simulink model "PTHS"  (R2020a)
settings: Solver=FixedStepAuto  StartTime=0.0  StopTime=10.0  FixedStep=1e-3  RelTol=1e-3  EnableMultiTasking=on
undefined symbols (not defined in the file): D0, D1, D10, D11, D12, D13, D2, D3, D4, D5, D6, D7, D8, D9, PTA0, PTA1, PTA2, PTB23, PTB9, PTC16, PTC17, PTC2, PTC3, PTC4, PTD0, PTD1, PTD2, PTD3
libraries: frdmk64flib x14
settings Model: ExtModeTrigDuration=5  Creator=iceca  LastModifiedBy=iceca
settings OptimizationCC: EnhancedBackFolding=on  PassReuseOutputArgsAs=Individual arguments  ZeroExternalMemoryAtStartup=off  ZeroInternalMemoryAtStartup=off  MaxStackSize=64  OptimizeBlockOrder=speed  DifferentSizesBufferReuse=on  OptimizationCustomize=off  EfficientTunableParamExpr=on
settings DebuggingCC: ParameterTunabilityLossMsg=error
settings HardwareCC: ProdBitPerPointer=32  ProdBitPerSizeT=32  ProdBitPerPtrDiffT=32  ProdLargestAtomicInteger=Long  ProdLargestAtomicFloat=Double  ProdWordSize=32  ProdHWDeviceType=ARM Compatible->ARM Cortex
settings SFSimCC: MATLABDynamicMemAlloc=off
settings RTWCC: SystemTargetFile=ert.tlc  HardwareBoard=NXP FRDM-K64F  TemplateMakefile=ert_default_tmf  Toolchain=GNU Tools for ARM Embedded Processors
settings CodeAppCC: ForceParamTrailComments=on  IgnoreCustomStorageClasses=off  OperatorAnnotations=on  SimulinkDataObjDesc=on  SFDataObjDesc=on  InsertBlockDesc=on

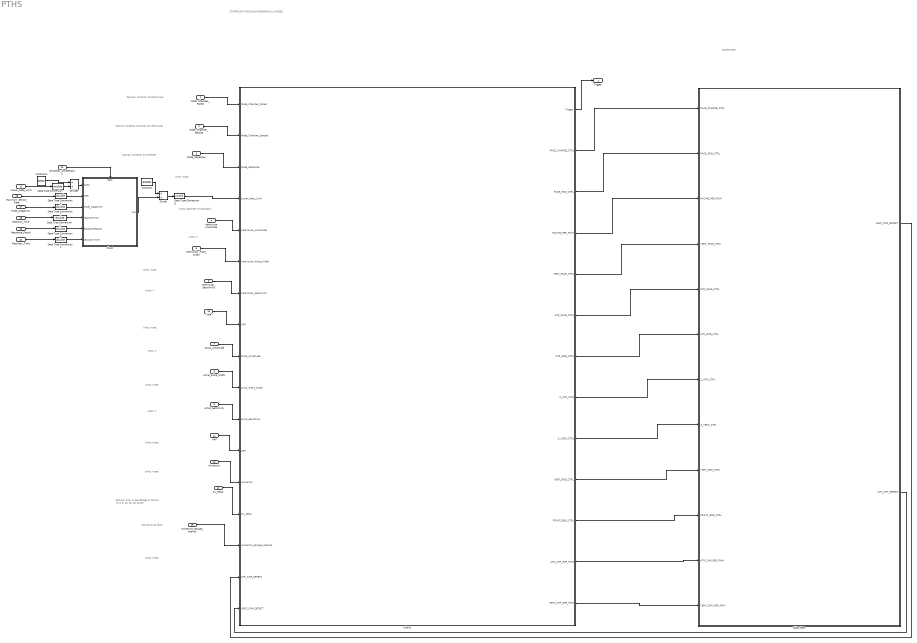
== system PTHS ==
  note: STATEFLOW: PACING and SENSING ALL MODES
  note: Units: msec
  note: Domain:true, false
  note: Domain: 0=None, 1=Atrial, 2=Ventricular
  note: Units: msec
  note: Units: V
  note: Units: V
  note: Units: msec
  note: Domain: OFF, or percentage
      | in the set (3, 6, 9, 12, 15, 18, 21,25)
  note: Units: msec
  note: Units: pace per minute(ppm)
  note: Units: msec
  note: Units: msec
  note: Domain: 1=Atrial, 2=Ventricular
  note: Units: V
  note: Units: msec
  note: Units: V
  note: HARDWARE
  note: Domain: 0=None, 2=Inhibited
  Mode_Chamber_Paced : Inport  OutDataTypeStr=uint8
  Mode_Chamber_Sensed : Inport  Port=2  OutDataTypeStr=uint8
  Mode_Response : Inport  Port=3  OutDataTypeStr=uint8
  Ventricular Amplitude : Inport  Port=4  OutDataTypeStr=uint8
  Ventricular_Pulse_Width : Inport  Port=5  OutDataTypeStr=uint16
  Ventricular_Sensiitivity : Inport  Port=6  OutDataTypeStr=uint8
  Atrial_Amplitude : Inport  Port=7  OutDataTypeStr=uint8
  Atrial_Pulse_Width : Inport  Port=8  OutDataTypeStr=uint16
  Atrial_Sensitivity : Inport  Port=9  OutDataTypeStr=uint8
  Hysterisis : Inport  Port=10  OutDataTypeStr=uint8
  Lower_Rate_Limit : Inport  Port=11  OutDataTypeStr=uint16
  AV_Delay : Inport  Port=12  OutDataTypeStr=uint16
  VRP : Inport  Port=13  OutDataTypeStr=uint16
  ARP : Inport  Port=14  OutDataTypeStr=uint16
  Hysterisis_Escape_Interval : Inport  Port=15  OutDataTypeStr=uint16
  Maximum_Sensor_Rate : Inport  Port=16  OutDataTypeStr=uint8
  Mode_Adaptivity : Inport  Port=17  OutDataTypeStr=uint8
  Reaction_Time : Inport  Port=18  OutDataTypeStr=uint8
  Response_Factor : Inport  Port=19  OutDataTypeStr=uint8
  Recovery_Time : Inport  Port=20  OutDataTypeStr=uint8
  Smoother_Acceleration : Inport  Port=21
  Chart : Stateflow chart  TreatAsAtomicUnit=on
      settings: PortSchema="{\"entries\":[{\"content\":{\"sides\":[{\"content\":{\"connectorIds\":[\"In6\"]},\"type\":\"ConnectorPlacement.EquallySpacedRectSide\",\"uuid\":\"5e590210-4b26-43ca-b410-899265592776\"},{\"content\":{\"connectorIds\":[],\"side\":\"RIGHT\"},\"type\":\"ConnectorPlacement.EquallySpacedRectSide\",\"uuid\":\"99d9f5d1-b5a6-4f8b-b4f2-efe260ebc8c4\"},{\"content\":{\"connectorIds\":[\"Out1\"],\"side\":\"TOP\"},\"type\":\"ConnectorPlacement.EquallySpacedRectSide\",\"uuid\":\"3c56162d-1f91-43ab-bf8d-9a1cf5be554c\"},{\"content\":{\"connectorIds\":[\"In1\",\"In2\",\"In7\",\"In4\",\"In3\",\"In5\"],\"side\":\"BOTTOM\"},\"type\":\"ConnectorPlacement.EquallySpacedRectSide\",\"uuid\":\"2e827a33-e1bf-40db-bbb6-314ece1f4eba\"}]},\"type\":\"ConnectorPlacement.EquallySpacedConnector\",\"uuid\":\"7a7dbe64-1607-48a8-bc2e-dcaf5b987588\"}],\"packageUris\":[\"http://schema.mathworks.com/mf0/Connector/19700101\"],\"version\":\"1.0\"}"
  Chart1 : Stateflow chart  TreatAsAtomicUnit=on
      settings: PortSchema="{\"entries\":[{\"content\":{\"sides\":[{\"content\":{\"connectorIds\":[\"In1\",\"In2\",\"In3\",\"In4\",\"In5\",\"In6\",\"In7\",\"In8\",\"In9\",\"In10\",\"In11\",\"In12\",\"In13\",\"In17\",\"In14\",\"In15\",\"In16\"]},\"type\":\"ConnectorPlacement.EquallySpacedRectSide\",\"uuid\":\"ef801456-a3d3-4c00-800f-18f55ff1f97a\"},{\"content\":{\"connectorIds\":[\"Out1\",\"Out2\",\"Out3\",\"Out4\",\"Out5\",\"Out6\",\"Out7\",\"Out8\",\"Out9\",\"Out10\",\"Out11\",\"Out12\",\"Out13\"],\"side\":\"RIGHT\"},\"type\":\"ConnectorPlacement.EquallySpacedRectSide\",\"uuid\":\"5ac52b61-bf48-4a4b-86f3-012ecfccb962\"},{\"content\":{\"connectorIds\":[],\"side\":\"TOP\"},\"type\":\"ConnectorPlacement.EquallySpacedRectSide\",\"uuid\":\"b91e78a1-d42c-4358-92cf-ad767f596c0a\"}]},\"type\":\"ConnectorPlacement.EquallySpacedConnector\",\"uuid\":\"810cd47a-6ba0-4b6e-85f5-59d182ca7955\"}],\"packageUris\":[\"http://schema.mathworks.com/mf0/Connector/19700101\"],\"version\":\"1.0\"}"
  Constant : Constant  Value=60000  SampleTime=-1
  Constant1 : Constant  Value=60000  SampleTime=-1
  Data Type Conversion{1..5,7} (6 alike) : DataTypeConversion  OutDataTypeStr=double
  Data Type Conversion8 : DataTypeConversion  OutDataTypeStr=uint16
  Divide : Product  Inputs=*/
  Divide1 : Product  Inputs=*/
  Subsystem : Subsystem
  Trigger : Outport
  wires:
  Chart1/1(Trigger) -> Trigger/1
  AV_Delay/1 -> Chart1/17(AV_Delay)
  Chart1/10(VENT_GND_CTRL) -> Subsystem/9(VENT_GND_CTRL)
  Chart1/12(ATR_CMP_REF_PWM) -> Subsystem/11(ATR_CMP_REF_PWM)
  Ventricular_Sensiitivity/1 -> Chart1/7(Ventricular_Sensitivity)
  Hysterisis_Escape_Interval/1 -> Chart1/14(Hysterisis_Escape_Interval)
  Chart1/5(VENT_PACE_CTRL) -> Subsystem/4(VENT_PACE_CTRL)
  Ventricular Amplitude/1 -> Chart1/5(Ventricular_Amplitude)
  VRP/1 -> Chart1/8(VRP)
  Chart1/13(VENT_CMP_REF_PWM) -> Subsystem/12(VENT_CMP_REF_PWM)
  Atrial_Amplitude/1 -> Chart1/9(Atrial_Amplitude)
  Chart1/6(ATR_PACE_CTRL) -> Subsystem/5(ATR_PACE_CTRL)
  Chart1/2(PACE_CHARGE_CTRL) -> Subsystem/1(PACE_CHARGE_CTRL)
  Atrial_Sensitivity/1 -> Chart1/11(Atrial_Sensitivity)
  Atrial_Pulse_Width/1 -> Chart1/10(Atrial_Pulse_Width)
  Mode_Response/1 -> Chart1/3(Mode_Response)
  Chart1/7(ATR_GND_CTRL) -> Subsystem/6(ATR_GND_CTRL)
  Mode_Chamber_Paced/1 -> Chart1/1(Mode_Chamber_Paced)
  Subsystem/1(VENT_CMP_DETECT) -> Chart1/15(ATR_CMP_DETECT)
  Chart1/11(FRONT_END_CTRL) -> Subsystem/10(FRONT_END_CTRL)
  Chart1/8(Z_ATR_CTRL) -> Subsystem/7(Z_ATR_CTRL)
  Chart1/3(PACE_GND_CTRL) -> Subsystem/2(PACE_GND_CTRL)
  Subsystem/2(ATR_CMP_DETECT) -> Chart1/16(VENT_CMP_DETECT)
  ARP/1 -> Chart1/12(ARP)
  Ventricular_Pulse_Width/1 -> Chart1/6(Ventricular_Pulse_Width)
  Mode_Chamber_Sensed/1 -> Chart1/2(Mode_Chamber_Sensed)
  Chart1/9(Z_VENT_CTRL) -> Subsystem/8(Z_VENT_CTRL)
  Chart1/4(PACING_REF_PWM) -> Subsystem/3(PACING_REF_PWM)
  Hysterisis/1 -> Chart1/13(Hysterisis)
  Chart/1(LRL) -> Divide/2
  Lower_Rate_Limit/1 -> Data Type Conversion5/1
  Reaction_Time/1 -> Data Type Conversion2/1
  Data Type Conversion1/1 -> Chart/5(recoveryTime)
  Data Type Conversion7/1 -> Chart/7(Mode_Adaptivity)
  Data Type Conversion2/1 -> Chart/4(reactionTime)
  Constant/1 -> Divide/1
  Data Type Conversion5/1 -> Divide1/2
  Data Type Conversion8/1 -> Chart1/4(Lower_Rate_Limit)
  Mode_Adaptivity/1 -> Data Type Conversion7/1
  Data Type Conversion3/1 -> Chart/3(ResponseFactor)
  Divide/1 -> Data Type Conversion8/1
  Constant1/1 -> Divide1/1
  Divide1/1 -> Chart/1(OLRL)
  Data Type Conversion4/1 -> Chart/2(MSR)
  Response_Factor/1 -> Data Type Conversion3/1
  Recovery_Time/1 -> Data Type Conversion1/1
  Maximum_Sensor_Rate/1 -> Data Type Conversion4/1
  Smoother_Acceleration/1 -> Chart/6(data)

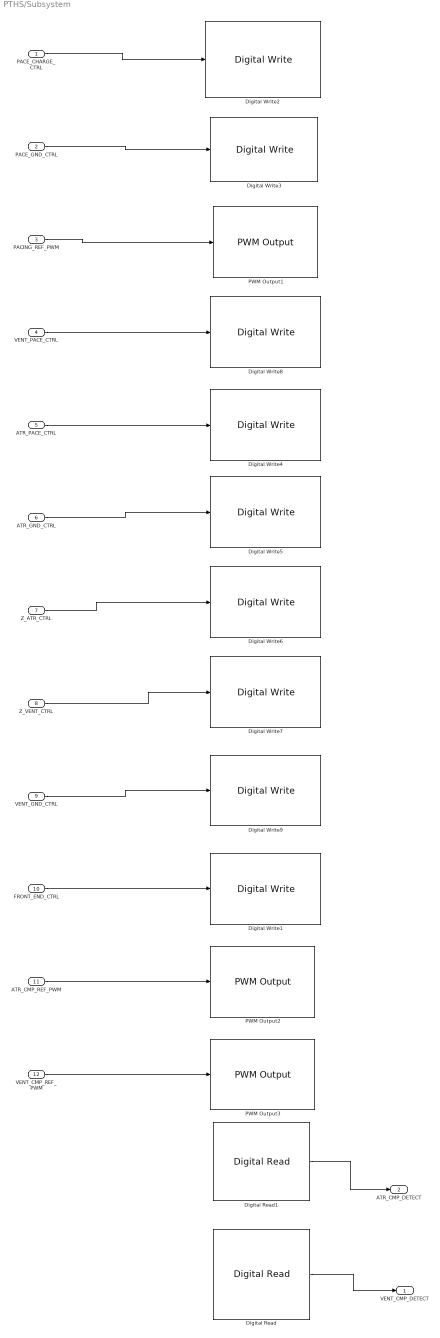
== system PTHS/Subsystem ==
  PACE_CHARGE_CTRL : Inport
  PACE_GND_CTRL : Inport  Port=2
  PACING_REF_PWM : Inport  Port=3
  VENT_PACE_CTRL : Inport  Port=4
  ATR_PACE_CTRL : Inport  Port=5
  ATR_GND_CTRL : Inport  Port=6
  Z_ATR_CTRL : Inport  Port=7
  Z_VENT_CTRL : Inport  Port=8
  VENT_GND_CTRL : Inport  Port=9
  FRONT_END_CTRL : Inport  Port=10
  ATR_CMP_REF_PWM : Inport  Port=11
  VENT_CMP_REF_PWM : Inport  Port=12
  Digital Read : frdmk64flib/Digital Read  Whichpin=PTC16 (D0)  SampleTime=-1
  Digital Read1 : frdmk64flib/Digital Read  Whichpin=PTC17 (D1)  SampleTime=-1
  Digital Write1 : frdmk64flib/Digital Write  Whichpin=PTD1 (D13)
  Digital Write2 : frdmk64flib/Digital Write  Whichpin=PTB9 (D2)
  Digital Write3 : frdmk64flib/Digital Write  Whichpin=PTD0 (D10)
  Digital Write4 : frdmk64flib/Digital Write  Whichpin=PTA0 (D8)
  Digital Write5 : frdmk64flib/Digital Write  Whichpin=PTD2 (D11)
  Digital Write6 : frdmk64flib/Digital Write  Whichpin=PTB23 (D4)
  Digital Write7 : frdmk64flib/Digital Write  Whichpin=PTC3 (D7)
  Digital Write8 : frdmk64flib/Digital Write  Whichpin=PTC4 (D9)
  Digital Write9 : frdmk64flib/Digital Write  Whichpin=PTD3 (D12)
  PWM Output1 : frdmk64flib/PWM Output  Whichpin=PTA2 (D5)  InitialFrequency=2000  InitialDutyCycle=0
  PWM Output2 : frdmk64flib/PWM Output  Whichpin=PTC2 (D6)  InitialFrequency=2000  InitialDutyCycle=0
  PWM Output3 : frdmk64flib/PWM Output  Whichpin=PTA1 (D3)  InitialFrequency=2000  InitialDutyCycle=0
  VENT_CMP_DETECT : Outport
  ATR_CMP_DETECT : Outport  Port=2
  wires:
  PACING_REF_PWM/1 -> PWM Output1/1
  VENT_GND_CTRL/1 -> Digital Write9/1
  PACE_GND_CTRL/1 -> Digital Write3/1
  ATR_GND_CTRL/1 -> Digital Write5/1
  ATR_CMP_REF_PWM/1 -> PWM Output2/1
  VENT_PACE_CTRL/1 -> Digital Write8/1
  Digital Read1/1 -> ATR_CMP_DETECT/1
  Digital Read/1 -> VENT_CMP_DETECT/1
  VENT_CMP_REF_PWM/1 -> PWM Output3/1
  Z_VENT_CTRL/1 -> Digital Write7/1
  Z_ATR_CTRL/1 -> Digital Write6/1
  PACE_CHARGE_CTRL/1 -> Digital Write2/1
  ATR_PACE_CTRL/1 -> Digital Write4/1
  FRONT_END_CTRL/1 -> Digital Write1/1

== stateflow chart PTHS/Chart ==
  state start
    exit:
    LRL = OLRL;
  state main
    entry:
    RateChange=ResponseFactor/4;
    %make sure LRL never exceeds MSR or goes below MSR
    LRL = max(OLRL, LRL);
    LRL=min(LRL, MSR);
  state Increasing
    entry:
    LRL=LRL+RateChange;
  state Constant
    entry:
    LRL=OLRL;
  state Decreasing
    entry:
    LRL=LRL-RateChange;
  (default) -> start
  start -> main : [OLRL>0 && OLRL<=2500]
  main -> Increasing [order 2] : [Mode_Adaptivity==1 && data>2.0 && LRL<MSR]
  Constant -> main
  Increasing -> main : [after(reactionTime,msec)]
  main -> Constant [order 3] : [Mode_Adaptivity==0]
  Decreasing -> main : [after(recoveryTime,msec)]
  main -> Decreasing [order 1] : [Mode_Adaptivity==1 && data<2.0 && LRL>OLRL]
  data: OLRL input; MSR input; ResponseFactor input; reactionTime input; recoveryTime input; data input; LRL output double; RateChange local; Mode_Adaptivity input

== stateflow chart PTHS/Chart1 ==
  state DUAL_MODES
    state A_PACING
      entry:
      PACE_CHARGE_CTRL = LOW;
      PACE_GND_CTRL = HIGH;
      VENT_PACE_CTRL = LOW;
      ATR_GND_CTRL =LOW;
      Z_ATR_CTRL = LOW;
      Z_VENT_CTRL = LOW;
      VENT_GND_CTRL = LOW;
      ATR_PACE_CTRL =HIGH;
    state V_CHARGING_A_DISCHARGING
      entry:
      %Charging c22
      ATR_PACE_CTRL=LOW;
      VENT_PACE_CTRL=LOW;
      PACING_REF_PWM=Ventricular_Amplitude;
      PACE_CHARGE_CTRL=HIGH;
      %Discharging Atrium
      PACE_GND_CTRL=HIGH;
      VENT_PACE_CTRL=LOW;
      Z_ATR_CTRL=LOW;
      Z_VENT_CTRL=LOW;
      ATR_PACE_CTRL=LOW;
      ATR_GND_CTRL=HIGH;
      VENT_GND_CTRL=LOW;
    state A_CHARGING_V_DISCHARGING
      entry:
      %charge atrium
      ATR_PACE_CTRL=LOW;
      VENT_PACE_CTRL=LOW;
      PACING_REF_PWM=Atrial_Amplitude;
      PACE_CHARGE_CTRL=HIGH;
      %discharge ventricle
      PACE_GND_CTRL=HIGH;
      VENT_PACE_CTRL=LOW;
      Z_ATR_CTRL=LOW;
      Z_VENT_CTRL=LOW;
      ATR_PACE_CTRL=LOW;
      ATR_GND_CTRL=LOW;
      VENT_GND_CTRL=HIGH;
      Atrial_Escape_Interval =Lower_Rate_Limit-AV_Delay;
      Trigger = HIGH;
    state V_PACING
      entry:
      PACE_CHARGE_CTRL = LOW;
      PACE_GND_CTRL = HIGH;
      ATR_PACE_CTRL = LOW;
      ATR_GND_CTRL =LOW;
      Z_ATR_CTRL = LOW;
      Z_VENT_CTRL = LOW;
      VENT_GND_CTRL = LOW;
      VENT_PACE_CTRL =HIGH;
    A_CHARGING_V_DISCHARGING -> A_PACING : [after(Atrial_Escape_Interval-Atrial_Pulse_Width-Ventricular_Pulse_Width, msec)]
    A_PACING -> V_CHARGING_A_DISCHARGING : [after(Atrial_Pulse_Width,msec)]
    V_CHARGING_A_DISCHARGING -> V_PACING : [after(AV_Delay,msec)]
  note: All inputs are integers and already processed. Hence the pins can be assigned to the inputs directly.
  state DECIDE_STATEFLOW
    entry:
    %Upon new cycle, trigger the parameter update
    Trigger=LOW;
    during:
    %During is reached when inputs are data stores are empty (zero),
    %such as before the any serial data is sent
    %(e.g. when model is first deployed to the board).
    %Continuously update the data stores by trigerring the update subsystem
    Trigger=~Trigger;
  state NON_DUAL_MODES
    state Charging_C23
      entry:
      ATR_PACE_CTRL   = LOW;
      VENT_PACE_CTRL = LOW;
      Trigger = HIGH;
    state Atrial_Charge
      entry:
      PACING_REF_PWM = Atrial_Amplitude;
    state Ventricular_Charge
      entry:
      PACING_REF_PWM = Ventricular_Amplitude;
    state Discharging_C21_and_Pace_Interval_Calculations
      entry:
      PACE_CHARGE_CTRL = HIGH;
      %Discharging C21
      PACE_GND_CTRL=HIGH;
      VENT_PACE_CTRL=LOW;
      Z_ATR_CTRL= LOW;
      Z_VENT_CTRL = LOW;
      ATR_PACE_CTRL = LOW;
      Pace_Interval = Lower_Rate_Limit;
      if Hysterisis == HIGH
      Pace_Interval = Pace_Interval + Hysterisis_Escape_Interval;
      end
    note: Pace_Interval is a local variable representing how long to wait (in msec) before pacing. It is updated along the stateflow, to acount for pulse widths, hysterisis and lower rate limit.
    state Atrial_Discharge
      entry:
      ATR_GND_CTRL= HIGH;
      VENT_GND_CTRL= LOW;
      Pace_Interval =Pace_Interval-Atrial_Pulse_Width;
    state Ventricular_Discharge
      entry:
      ATR_GND_CTRL = LOW;
      VENT_GND_CTRL = HIGH;
      Pace_Interval =Pace_Interval -Ventricular_Pulse_Width;
    state Atrial_Sensing
      entry:
      FRONT_END_CTRL = HIGH;
      ATR_CMP_REF_PWM= Atrial_Sensitivity;
    state Ventricular_Sensing
      entry:
      FRONT_END_CTRL = HIGH;
      VENT_CMP_REF_PWM = Ventricular_Sensitivity;
    state No_Natural_Activity_Sensed
      entry:
      FRONT_END_CTRL = HIGH;
    state Pacing_Begin
      entry:
      PACE_CHARGE_CTRL = LOW;
      PACE_GND_CTRL = HIGH;
    state Ventricular_Pacing
      entry:
      ATR_PACE_CTRL = LOW;
    state Atrial_Pacing
      entry:
      VENT_PACE_CTRL = LOW;
    state Pacing
      entry:
      ATR_GND_CTRL =LOW;
      Z_ATR_CTRL = LOW;
      Z_VENT_CTRL = LOW;
      VENT_GND_CTRL = LOW;
    state Vent_Pacing_2
      entry:
      VENT_PACE_CTRL =HIGH;
    state Atrial_Pacing_2
      entry:
      ATR_PACE_CTRL =HIGH;
    Charging_C23 -> Atrial_Charge [order 2] : [Mode_Chamber_Paced==1]
    Charging_C23 -> Ventricular_Charge [order 1] : [Mode_Chamber_Paced==2]
    Atrial_Charge -> Discharging_C21_and_Pace_Interval_Calculations
    Ventricular_Charge -> Discharging_C21_and_Pace_Interval_Calculations
    Discharging_C21_and_Pace_Interval_Calculations -> Ventricular_Discharge [order 2] : [Mode_Chamber_Paced==2]
    Discharging_C21_and_Pace_Interval_Calculations -> Atrial_Discharge [order 1] : [Mode_Chamber_Paced==1]
    Atrial_Discharge -> Atrial_Sensing [order 2] : [Mode_Chamber_Sensed==1]
    Atrial_Discharge -> No_Natural_Activity_Sensed [order 1] : [Mode_Chamber_Sensed==0 && after(Pace_Interval, msec)]
    Ventricular_Discharge -> No_Natural_Activity_Sensed [order 2] : [Mode_Chamber_Sensed==0 && after(Pace_Interval, msec)]
    Ventricular_Discharge -> Ventricular_Sensing [order 1] : [Mode_Chamber_Sensed==2]
    Atrial_Sensing -> No_Natural_Activity_Sensed [order 1] : [after(Pace_Interval,msec)]
    Ventricular_Sensing -> No_Natural_Activity_Sensed [order 1] : [after(Pace_Interval,msec)]
    No_Natural_Activity_Sensed -> Pacing_Begin
    Pacing_Begin -> Ventricular_Pacing [order 1] : [Mode_Chamber_Paced==2]
    Pacing_Begin -> Atrial_Pacing [order 2] : [Mode_Chamber_Paced==1]
    Atrial_Pacing -> Pacing
    Ventricular_Pacing -> Pacing
    Pacing -> Atrial_Pacing_2 [order 2] : [Mode_Chamber_Paced==1]
    Pacing -> Vent_Pacing_2 [order 1] : [Mode_Chamber_Paced==2]
  note: Phase 1:
      | Charging Capacitors
  note: ----------------------------------------------------------------------------------
  note: Phase 2:
      | Discharging Capacitors
  note: ---------------------------------------------------------------------------------
  note: Phase 3:
      | Sensing
  note: ----------------------------------------------------------------------------------
  note: Phase 4:
      | Pacing
  DECIDE_STATEFLOW -> A_CHARGING_V_DISCHARGING [order 1] : [Mode_Chamber_Paced==3]
  V_PACING -> DECIDE_STATEFLOW : [after(Ventricular_Pulse_Width,msec)]
  (default) -> DECIDE_STATEFLOW
  Vent_Pacing_2 -> DECIDE_STATEFLOW : [after(Ventricular_Pulse_Width,msec)]
  Atrial_Pacing_2 -> DECIDE_STATEFLOW : [after(Atrial_Pulse_Width,msec)]
  Ventricular_Sensing -> DECIDE_STATEFLOW [order 2] : [Mode_Response==2 &&  VENT_CMP_DETECT==true && after(VRP, msec)]
  Atrial_Sensing -> DECIDE_STATEFLOW [order 2] : [Mode_Response==2 && after(ARP, msec) && ATR_CMP_DETECT==HIGH]
  DECIDE_STATEFLOW -> Charging_C23 [order 2] : [Mode_Chamber_Paced==2 || Mode_Chamber_Paced==1]
  data: Trigger output; Mode_Chamber_Paced input; Mode_Chamber_Sensed input; Mode_Response input; PACE_CHARGE_CTRL output; PACE_GND_CTRL output; PACING_REF_PWM output; VENT_PACE_CTRL output; ATR_PACE_CTRL output; ATR_GND_CTRL output; Z_ATR_CTRL output; Z_VENT_CTRL output; VENT_GND_CTRL output; Lower_Rate_Limit input; HIGH local boolean =true; LOW local boolean =false; Ventricular_Amplitude input; Ventricular_Pulse_Width input; Ventricular_Sensitivity input; VRP input; Atrial_Amplitude input; Atrial_Pulse_Width input; Atrial_Sensitivity input; ARP input; FRONT_END_CTRL output; ATR_CMP_REF_PWM output; VENT_CMP_REF_PWM output; Hysterisis input; Hysterisis_Escape_Interval input; ATR_CMP_DETECT input; VENT_CMP_DETECT input; Pace_Interval local; AV_Delay input; Atrial_Escape_Interval local
